simulink model "ee_dyn_check_sim"  (R2022a)
settings: Solver=VariableStepAuto  StartTime=0.0  StopTime=5  RelTol=1e-3
values from neighbouring files (symbols this model uses):
  N = 12    [pred_val_data.mat]
  tau = predLogsout.getElement('tau').Values    [testNmpcPred.m]
settings Model: Creator=charl  LastModifiedBy=charl

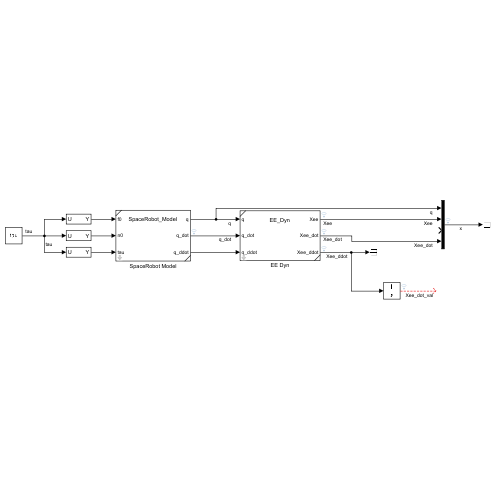
[thumbnail: Simulink's stored preview of the top-level diagram]
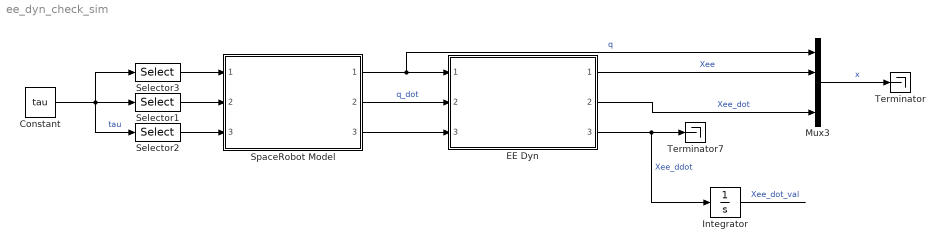
== system ee_dyn_check_sim ==
  Constant : Constant  Value=tau
  EE Dyn : Subsystem  ReferencedSubsystem=EE_Dyn  spaceRobot=sr
  Integrator : Integrator  InitialCondition=zeros(6, 1)
  Mux3 : Mux
  Selector1 : Selector  IndexOptions=Index vector (dialog)  Indices=[4:6]  OutputSizes=1
  Selector2 : Selector  IndexOptions=Index vector (dialog)  Indices=[7:N]  OutputSizes=1
  Selector3 : Selector  IndexOptions=Index vector (dialog)  Indices=[1:3]  OutputSizes=1
  SpaceRobot Model : Subsystem  ReferencedSubsystem=SpaceRobot_Model  spaceRobot=sr  jointCstr=off  q_0=q0  q_dot_0=q_dot_0
  Terminator : Terminator
  Terminator7 : Terminator
  wires:
  SpaceRobot Model/3 -> EE Dyn/3
  EE Dyn/3 -> Integrator/1, Terminator7/1  "Xee_ddot"
  EE Dyn/1 -> Mux3/2  "Xee"
  Selector2/1 -> SpaceRobot Model/3
  SpaceRobot Model/1 -> EE Dyn/1, Mux3/1  "q"
  Mux3/1 -> Terminator/1  "x"
  Integrator/1 -> ?  "Xee_dot_val"
  Selector3/1 -> SpaceRobot Model/1
  Constant/1 -> Selector2/1, Selector1/1, Selector3/1  "tau"
  SpaceRobot Model/2 -> EE Dyn/2  "q_dot"
  Selector1/1 -> SpaceRobot Model/2
  EE Dyn/2 -> Mux3/4  "Xee_dot"
